simulink model "Main"  (R2020b)
settings: Solver=FixedStepAuto  StartTime=0.0  StopTime=40  FixedStep=0.01  RelTol=1e-3
settings Model: Creator=kaebi  LastModifiedBy=kaebi
settings OptimizationCC: DefaultParameterBehavior=Inlined  LocalBlockOutputs=off
settings RTWCC: Description=TwinCAT GRT Target  SystemTargetFile=TwinCatGrt.tlc  GenCodeOnly=on  TemplateMakefile=tcgrt_msbuild.tmf  TargetLang=C++
settings STFCustomTargetCC: TargetLangStandard=C++03 (ISO)  ConcurrentExecutionCompliant=off  CombineOutputUpdateFcns=on  CodeInterfacePackaging=Reusable function  GRTInterface=off  GenerateAllocFcn=on  SystemTargetFile=TwinCatGrt.tlc
settings GRTTargetCC: TargetLangStandard=C++03 (ISO)  ParMdlRefBuildCompliant=off  CompOptLevelCompliant=off  ConcurrentExecutionCompliant=off  MatFileLogging=off  CodeInterfacePackaging=Reusable function  GenerateAllocFcn=on  UseToolchainInfoCompliant=off  ExtModeMexFile=TcExtModeClient

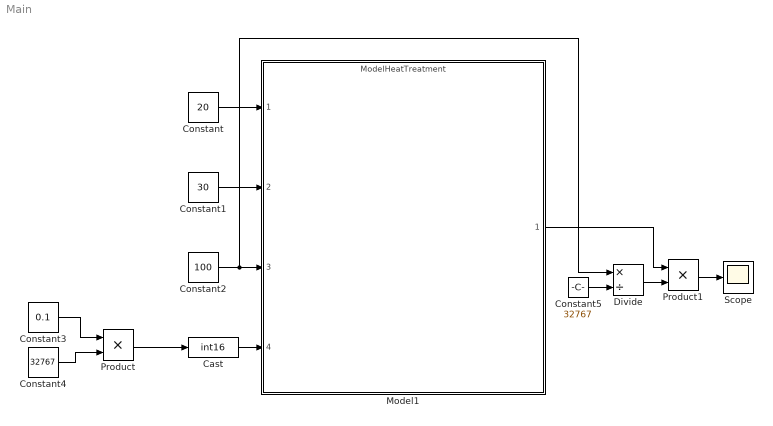
== system Main ==
  Cast : DataTypeConversion  OutDataTypeStr=int16
  Constant : Constant  Value=20
  Constant1 : Constant  Value=30
  Constant2 : Constant  Value=100
  Constant3 : Constant  Value=0.1
  Constant4 : Constant  Value=32767
  Constant5 : Constant  Value=32767
  Divide : Product  Inputs=*/
  Model1 : ModelReference  ModelNameDialog=ModelHeatTreatment.slx  SimulationMode=Normal  ModelReferenceVersion=1.28
  Product : Product
  Product1 : Product
  Scope : Scope
  wires:
  Constant1/1 -> Model1/2
  Constant2/1 -> Divide/1, Model1/3
  Product/1 -> Cast/1
  Constant3/1 -> Product/1
  Constant4/1 -> Product/2
  Cast/1 -> Model1/4
  Divide/1 -> Product1/2
  Model1/1 -> Product1/1
  Product1/1 -> Scope/1
  Constant5/1 -> Divide/2
  Constant/1 -> Model1/1
